simulink model "rl_3tank"  (R2023a)
settings: Solver=VariableStepAuto  StartTime=0.0  StopTime=1000  RelTol=1e-3
undefined symbols (not defined in the file or in its folder): A, az1, az2, az3, g, H_star1, H_star2, Qmax, Sn
libraries: rllib x1
settings Model: Creator=empg0  LastModifiedBy=empg0
settings SolverCC: ZeroCrossAlgorithm=Adaptive
settings DebuggingCC: IgnoredZcDiagnostic=none

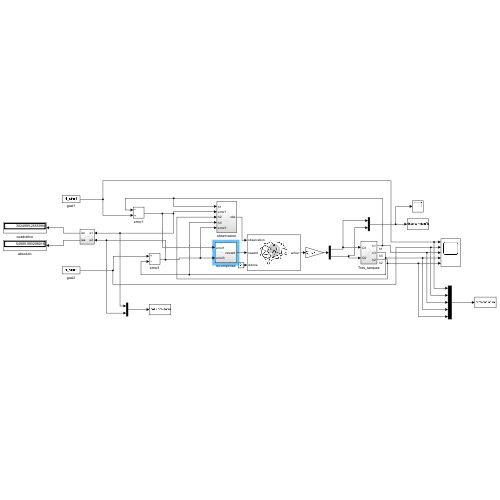
[thumbnail: Simulink's stored preview of the top-level diagram]
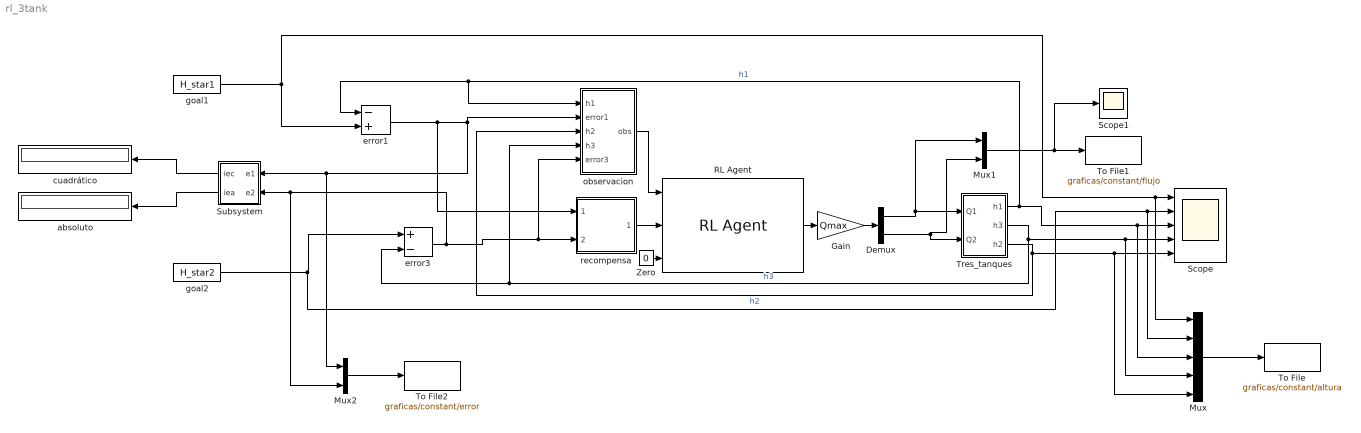
== system rl_3tank ==
  Demux : Demux  Outputs=2
  Gain : Gain  Gain=Qmax
  Mux : Mux  Inputs=5
  Mux1 : Mux  Inputs=2
  Mux2 : Mux  Inputs=2
  RL Agent : rllib/RL Agent  Agent=agent  ExternalActionAsInput=off  ProvideLastAction=off  ProvideCumRwd=off  TreatAsDirectFeedthrough=on  UseStrictObservationDataTypes=off
  Scope : Scope  NumInputPorts=5
  Scope1 : Scope
  Subsystem : Subsystem
  To File : ToFile  Filename=graficas/constant/altura  MatrixName=altura  SampleTime=0.5
  To File1 : ToFile  Filename=graficas/constant/flujo  MatrixName=flujo  SampleTime=0.5
  To File2 : ToFile  Filename=graficas/constant/error  MatrixName=error  SampleTime=0.5
  Tres_tanques : Subsystem
  Zero : Constant  Value=0  OutDataTypeStr=Inherit: Inherit via back propagation
  absoluto : Display
  cuadrático : Display
  error1 : Sum  Inputs=-+
  error3 : Sum  Inputs=+-
  goal1 : Constant  Value=H_star1
  goal2 : Constant  Value=H_star2
  observacion : Subsystem
  recompensa : Subsystem
  wires:
  Zero/1 -> RL Agent/3
  recompensa/1(reward) -> RL Agent/2
  observacion/1(obs) -> RL Agent/1
  Tres_tanques/1(h1) -> Mux/3, Scope/3, observacion/1(h1), error1/1  "h1"
  error1/1 -> Mux2/1, Subsystem/1(e1), observacion/2(error1), recompensa/1(error1)
  goal2/1 -> Mux/2, Scope/2, error3/1
  Tres_tanques/3(h2) -> observacion/3(h2), Mux/5, Scope/5  "h2"
  error3/1 -> Mux2/2, Subsystem/2(e2), observacion/5(error3), recompensa/2(error3)
  Tres_tanques/2(h3) -> observacion/4(h3), error3/2, Mux/4, Scope/4  "h3"
  Demux/2 -> Tres_tanques/2(Q2), Mux1/2
  goal1/1 -> error1/2, Mux/1, Scope/1
  Subsystem/1(iec) -> cuadrático/1
  Mux/1 -> To File/1
  Mux1/1 -> Scope1/1, To File1/1
  Mux2/1 -> To File2/1
  Subsystem/2(iea) -> absoluto/1
  RL Agent/1 -> Gain/1
  Gain/1 -> Demux/1
  Demux/1 -> Tres_tanques/1(Q1), Mux1/1

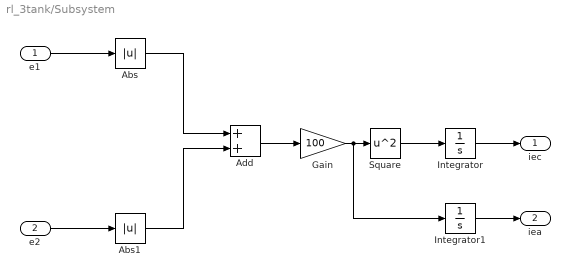
== system rl_3tank/Subsystem ==
  e1 : Inport
  e2 : Inport  Port=2
  Abs : Abs  SaturateOnIntegerOverflow=off
  Abs1 : Abs  SaturateOnIntegerOverflow=off
  Add : Sum
  Gain : Gain  Gain=100
  Integrator : Integrator
  Integrator1 : Integrator
  Square : Math  Operator=square
  iec : Outport
  iea : Outport  Port=2
  wires:
  Abs/1 -> Add/1
  Square/1 -> Integrator/1
  Integrator/1 -> iec/1
  e2/1 -> Abs1/1
  Abs1/1 -> Add/2
  e1/1 -> Abs/1
  Gain/1 -> Integrator1/1, Square/1
  Add/1 -> Gain/1
  Integrator1/1 -> iea/1

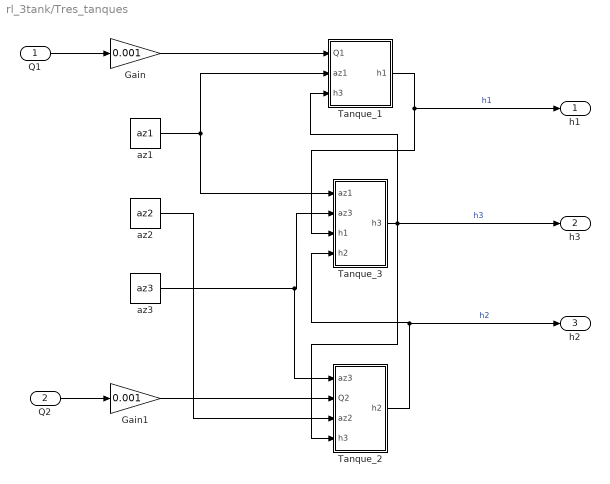
== system rl_3tank/Tres_tanques ==
  Q1 : Inport
  Q2 : Inport  Port=2
  Gain : Gain  Gain=0.001
  Gain1 : Gain  Gain=0.001
  Tanque_1 : Subsystem
  Tanque_2 : Subsystem
  Tanque_3 : Subsystem
  az1 : Constant  Value=az1
  az2 : Constant  Value=az2
  az3 : Constant  Value=az3
  h1 : Outport
  h3 : Outport  Port=2
  h2 : Outport  Port=3
  wires:
  Tanque_2/1(h2) -> Tanque_3/4(h2), h2/1  "h2"
  Tanque_1/1(h1) -> Tanque_3/3(h1), h1/1  "h1"
  Gain1/1 -> Tanque_2/2(Q2)
  Tanque_3/1(h3) -> Tanque_2/4(h3), h3/1, Tanque_1/3(h3)  "h3"
  az3/1 -> Tanque_2/1(az3), Tanque_3/2(az3)
  az1/1 -> Tanque_3/1(az1), Tanque_1/2(az1)
  az2/1 -> Tanque_2/3(az2)
  Gain/1 -> Tanque_1/1(Q1)
  Q1/1 -> Gain/1
  Q2/1 -> Gain1/1

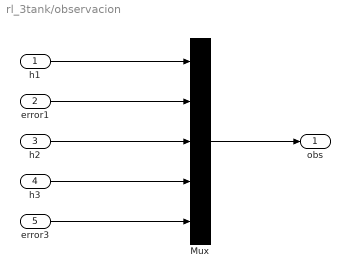
== system rl_3tank/observacion ==
  h1 : Inport
  error1 : Inport  Port=2
  h2 : Inport  Port=3
  h3 : Inport  Port=4
  error3 : Inport  Port=5
  Mux : Mux  Inputs=5
  obs : Outport
  wires:
  Mux/1 -> obs/1
  error1/1 -> Mux/2
  h1/1 -> Mux/1
  h2/1 -> Mux/3
  h3/1 -> Mux/4
  error3/1 -> Mux/5

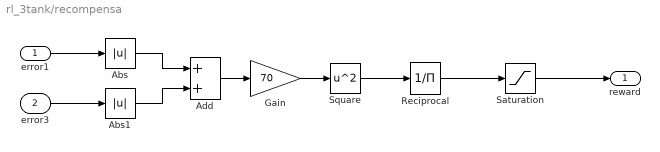
== system rl_3tank/recompensa ==
  error1 : Inport
  error3 : Inport  Port=2
  Abs : Abs  SaturateOnIntegerOverflow=off
  Abs1 : Abs  SaturateOnIntegerOverflow=off
  Add : Sum
  Gain : Gain  Gain=70
  Reciprocal : Product  Inputs=/
  Saturation : Saturate  UpperLimit=3000  LowerLimit=0
  Square : Math  Operator=square
  reward : Outport
  wires:
  error1/1 -> Abs/1
  error3/1 -> Abs1/1
  Abs/1 -> Add/1
  Abs1/1 -> Add/2
  Square/1 -> Reciprocal/1
  Reciprocal/1 -> Saturation/1
  Saturation/1 -> reward/1
  Add/1 -> Gain/1
  Gain/1 -> Square/1

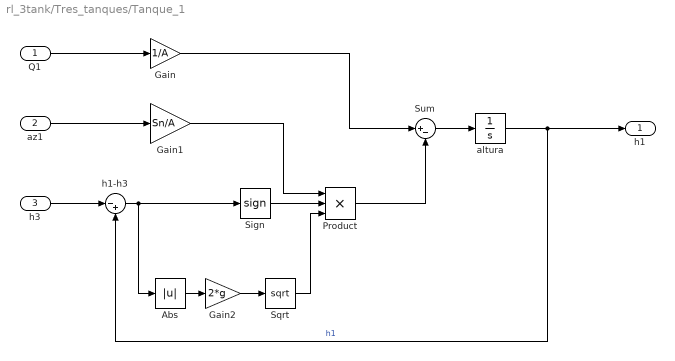
== system rl_3tank/Tres_tanques/Tanque_1 ==
  Q1 : Inport
  az1 : Inport  Port=2
  h3 : Inport  Port=3
  Abs : Abs  SaturateOnIntegerOverflow=off
  Gain : Gain  Gain=1/A
  Gain1 : Gain  Gain=Sn/A
  Gain2 : Gain  Gain=2*g
  Product : Product  Inputs=3
  Sign : Signum
  Sqrt : Sqrt
  Sum : Sum  Inputs=|+-
  altura : Integrator  LimitOutput=on  UpperSaturationLimit=0.62  LowerSaturationLimit=0
  h1-h3 : Sum  Inputs=|-+
  h1 : Outport
  wires:
  h3/1 -> h1-h3/1
  Sum/1 -> altura/1
  Gain2/1 -> Sqrt/1
  Gain1/1 -> Product/1
  Sqrt/1 -> Product/3
  Sign/1 -> Product/2
  h1-h3/1 -> Abs/1, Sign/1
  Q1/1 -> Gain/1
  az1/1 -> Gain1/1
  altura/1 -> h1/1, h1-h3/2  "h1"
  Product/1 -> Sum/2
  Gain/1 -> Sum/1
  Abs/1 -> Gain2/1

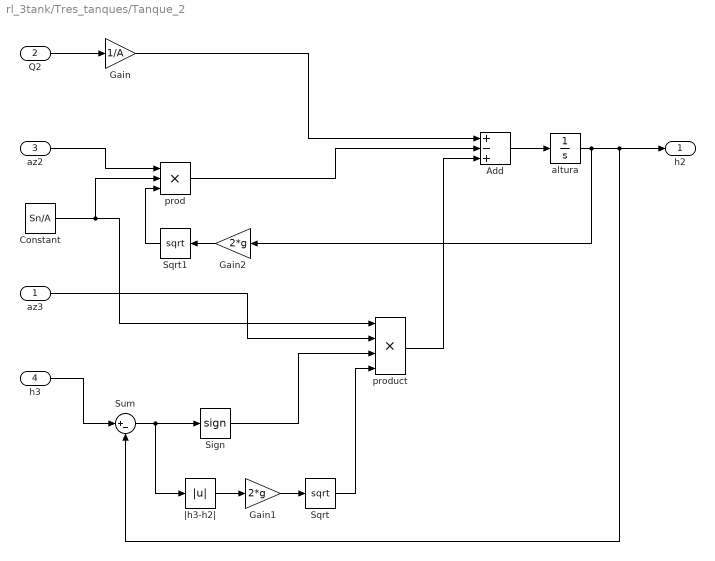
== system rl_3tank/Tres_tanques/Tanque_2 ==
  az3 : Inport
  Q2 : Inport  Port=2
  az2 : Inport  Port=3
  h3 : Inport  Port=4
  Add : Sum  Inputs=+-+
  Constant : Constant  Value=Sn/A
  Gain : Gain  Gain=1/A
  Gain1 : Gain  Gain=2*g
  Gain2 : Gain  Gain=2*g
  Sign : Signum
  Sqrt : Sqrt
  Sqrt1 : Sqrt
  Sum : Sum  Inputs=|+-
  altura : Integrator  LimitOutput=on  UpperSaturationLimit=0.62  LowerSaturationLimit=0
  prod : Product  Inputs=3
  product : Product  Inputs=4
  |h3-h2| : Abs  SaturateOnIntegerOverflow=off
  h2 : Outport
  wires:
  |h3-h2|/1 -> Gain1/1
  prod/1 -> Add/2
  product/1 -> Add/3
  Add/1 -> altura/1
  Gain/1 -> Add/1
  Constant/1 -> product/1, prod/2
  Gain1/1 -> Sqrt/1
  Sum/1 -> |h3-h2|/1, Sign/1
  az2/1 -> prod/1
  az3/1 -> product/2
  Sqrt1/1 -> prod/3
  Sqrt/1 -> product/4
  Sign/1 -> product/3
  h3/1 -> Sum/1
  altura/1 -> Gain2/1, h2/1, Sum/2
  Gain2/1 -> Sqrt1/1
  Q2/1 -> Gain/1

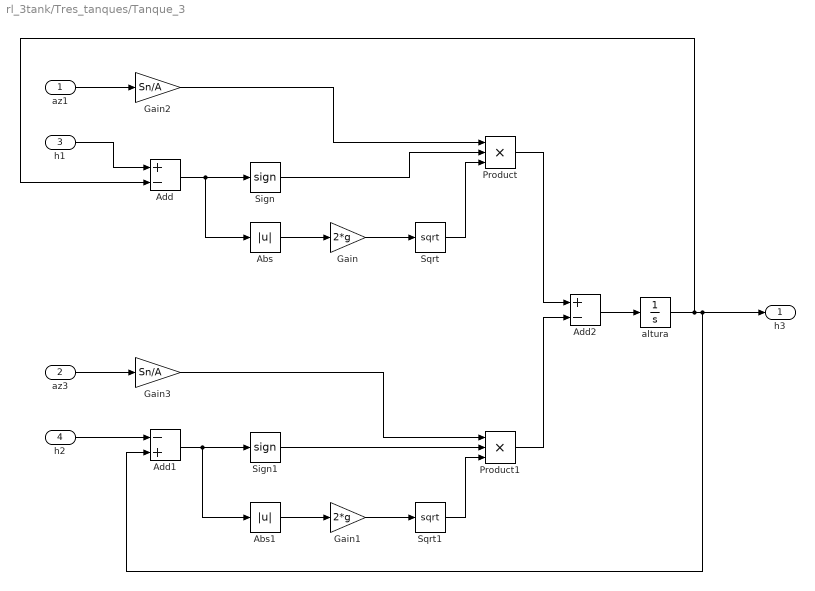
== system rl_3tank/Tres_tanques/Tanque_3 ==
  az1 : Inport
  az3 : Inport  Port=2
  h1 : Inport  Port=3
  h2 : Inport  Port=4
  Abs : Abs  SaturateOnIntegerOverflow=off
  Abs1 : Abs  SaturateOnIntegerOverflow=off
  Add : Sum  Inputs=+-
  Add1 : Sum  Inputs=-+
  Add2 : Sum  Inputs=+-
  Gain : Gain  Gain=2*g
  Gain1 : Gain  Gain=2*g
  Gain2 : Gain  Gain=Sn/A
  Gain3 : Gain  Gain=Sn/A
  Product : Product  Inputs=3
  Product1 : Product  Inputs=3
  Sign : Signum
  Sign1 : Signum
  Sqrt : Sqrt
  Sqrt1 : Sqrt
  altura : Integrator  LimitOutput=on  UpperSaturationLimit=0.62  LowerSaturationLimit=0
  h3 : Outport
  wires:
  Add2/1 -> altura/1
  Gain3/1 -> Product1/1
  az1/1 -> Gain2/1
  Gain1/1 -> Sqrt1/1
  Add1/1 -> Abs1/1, Sign1/1
  h1/1 -> Add/1
  az3/1 -> Gain3/1
  altura/1 -> h3/1, Add1/2, Add/2
  Abs1/1 -> Gain1/1
  Add/1 -> Abs/1, Sign/1
  Abs/1 -> Gain/1
  Sqrt1/1 -> Product1/3
  Sign/1 -> Product/2
  Product1/1 -> Add2/2
  Gain2/1 -> Product/1
  Sqrt/1 -> Product/3
  Sign1/1 -> Product1/2
  Gain/1 -> Sqrt/1
  h2/1 -> Add1/1
  Product/1 -> Add2/1
